simulink model "test_ps_helium_X"  (R2016a)
settings: Solver=VariableStepAuto  StartTime=0.0  StopTime=1000  RelTol=1e-3
libraries: simCryogenics_lib x18, nesl_utility x11
settings Model: Creator=FB229602  LastModifiedBy=FB229602
settings GRTTargetCC: GeneratePreprocessorConditionals=Use local settings
settings SimscapeCC: SimscapeLogType=all  SimscapeLogOpenViewer=on  SimscapeLogLimitData=off

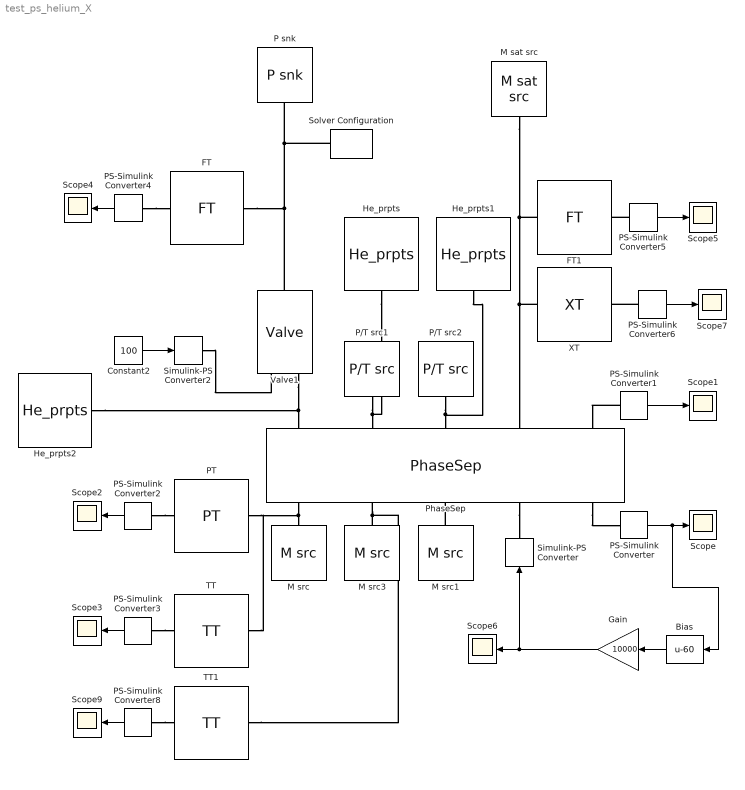
== system test_ps_helium_X ==
  Bias : Bias  Bias=-60
  Constant2 : Constant  Value=100
  FT : simCryogenics_lib/Sensors/FT
  FT1 : simCryogenics_lib/Sensors/FT
  Gain : Gain  Gain=10000
  He_prpts : simCryogenics_lib/Utilities/He_prpts  P_min=0.2 bar  T_min=1 K  T_max=100 K  P_max=50 bar  Mol=4.0026 * (10 ^ (- 3)) kg/mol
  He_prpts1 : simCryogenics_lib/Utilities/He_prpts  P_min=0.2 bar  T_min=1 K  T_max=100 K  P_max=50 bar  Mol=4.0026 * (10 ^ (- 3)) kg/mol
  He_prpts2 : simCryogenics_lib/Utilities/He_prpts  P_min=0.2 bar  T_min=1 K  T_max=100 K  P_max=50 bar  Mol=4.0026 * (10 ^ (- 3)) kg/mol
  M sat src : simCryogenics_lib/Sources_Sinks/M sat src  M=0.1 kg/s  Xmix=0.5
  M src : simCryogenics_lib/Sources_Sinks/M src  M=0 kg/s
  M src1 : simCryogenics_lib/Sources_Sinks/M src  M=0.05 kg/s
  M src3 : simCryogenics_lib/Sources_Sinks/M src  M=0.05 kg/s
  P snk : simCryogenics_lib/Sources_Sinks/P snk  P=1.05 bar
  P/T src1 : simCryogenics_lib/Sources_Sinks/P//T src  P=5 bar  T=5 K
  P/T src2 : simCryogenics_lib/Sources_Sinks/P//T src  P=5 bar  T=5 K
  PS-Simulink Converter{,1..6,8} (8 alike) : nesl_utility/PS-Simulink Converter  PhysicalDomain=network_engine_domain  SubClassName=ps_output  LeftPortType=input  RightPortType=output  PseudoPeriodic=off  Frequencies=[]  Unit=1  AffineConversion=off
  PT : simCryogenics_lib/Sensors/PT
  PhaseSep : simCryogenics_lib/Elements/PhaseSep  Ideal1=1  DeltaT1=0.05 K  N1=10  h1=400 W/K  Ideal2=1  DeltaT2=0.05 K  N2=10  h2=400 W/K  hmax=1.5 m  S=0.2 m^2  P0=1.2 bar  h0=62
  Scope{,1..7,9} (9 alike) : Scope
  Simulink-PS Converter : nesl_utility/Simulink-PS Converter  PhysicalDomain=network_engine_domain  SubClassName=ps_input  LeftPortType=input  RightPortType=output  PseudoPeriodic=off  Frequencies=[]  NoiseDistribution=none  NoiseParameters=[]  Unit=1  AffineConversion=off  InputFiltering=off  SimscapeFilterOrder=1  InputFilterTimeConstant=0.001  UdotUserProvided=1
  Simulink-PS Converter2 : nesl_utility/Simulink-PS Converter  PhysicalDomain=network_engine_domain  SubClassName=ps_input  LeftPortType=input  RightPortType=output  PseudoPeriodic=off  Frequencies=[]  NoiseDistribution=none  NoiseParameters=[]  Unit=1  AffineConversion=off  InputFiltering=off  SimscapeFilterOrder=1  InputFilterTimeConstant=0.001  UdotUserProvided=1
  Solver Configuration : nesl_utility/Solver Configuration  PhysicalDomain=network_engine_domain  SubClassName=solver  LeftPortType=input  RightPortType=generic  Accelerate=off  Tones=[]  Harmonics=[]  SimulateNoise=off  Profile=off  UseLocalSampling=off  EnableSwitchedLinearOptims=on  FrequencyDomain=off  UseCCode=off  RelTol=0.001  AbsTol=1e-06  MinStep=1e-09  ToWorkspace=off  RevertToSquareIcSolve=off  NumHomotopyIterations=100  PhasorMode=off  PhasorModeNumHarmonics=1  OverrideAbsTol=off  DoDC=off  ResidualTolerance=1e-09  UseLocalSolver=off  LocalSolverChoice=NE_BACKWARD_EULER_ADVANCER  LocalSolverSampleTime=0.001  DoFixedCost=off  MaxNonlinIter=3  MaxModeIter=2  LinearAlgebra=Sparse  DelaysMemoryBudget=1024  AutomaticFiltering=on  FilteringTimeConstant=0.001
  TT : simCryogenics_lib/Sensors/TT
  TT1 : simCryogenics_lib/Sensors/TT
  Valve1 : simCryogenics_lib/Elements/Valve  CVmax=100  ControlInputMin=0  ControlInputMax=100  Xt=0.86  Rv=10  lin_v=0  lim_v=0  K=2.4e-5 m^1.50000*kg^0.50000/s/bar^0.50000  Cmd_specify=off  Cmd_priority=None  Cmd=0  gamma_specify=off  gamma_priority=None  gamma=0  rho_specify=off  rho_priority=None  rho=0 kg/m^3  Xc_specify=off  Xc_priority=None  Xc=0  X_specify=off  X_priority=None  X=0  Y_specify=off  Y_priority=None  Y=0  CV_specify=off  CV_priority=None  CV=0
  XT : simCryogenics_lib/Sensors/XT
  wires:
  Gain/1 -> Simulink-PS Converter/1, Scope6/1
  PS-Simulink Converter/1 -> Bias/1, Scope/1
  PS-Simulink Converter1/1 -> Scope1/1
  Constant2/1 -> Simulink-PS Converter2/1
  PS-Simulink Converter2/1 -> Scope2/1
  PS-Simulink Converter3/1 -> Scope3/1
  PS-Simulink Converter4/1 -> Scope4/1
  PS-Simulink Converter5/1 -> Scope5/1
  Bias/1 -> Gain/1
  PS-Simulink Converter6/1 -> Scope7/1
  PS-Simulink Converter8/1 -> Scope9/1
  connections:
  PhaseSep/RConn1 -- TT/LConn1 -- PT/LConn1 -- M src/RConn1
  Valve1/RConn1 -- FT/LConn1 -- P snk/RConn1 -- Solver Configuration/RConn1
  FT1/LConn1 -- XT/LConn1 -- PhaseSep/LConn4 -- M sat src/RConn1
  M src3/RConn1 -- TT1/LConn1 -- PhaseSep/RConn2
  M src1/RConn1 -- PhaseSep/RConn3
  PhaseSep/RConn4 -- Simulink-PS Converter/RConn1
  PhaseSep/RConn5 -- PS-Simulink Converter/LConn1
  PS-Simulink Converter1/LConn1 -- PhaseSep/LConn5
  Valve1/LConn2 -- He_prpts2/RConn1 -- PhaseSep/LConn1
  Simulink-PS Converter2/RConn1 -- Valve1/LConn1
  PS-Simulink Converter2/LConn1 -- PT/RConn1
  P/T src1/RConn1 -- He_prpts/RConn1 -- PhaseSep/LConn2
  P/T src2/RConn1 -- He_prpts1/RConn1 -- PhaseSep/LConn3
  PS-Simulink Converter3/LConn1 -- TT/RConn1
  PS-Simulink Converter4/LConn1 -- FT/RConn1
  PS-Simulink Converter5/LConn1 -- FT1/RConn1
  PS-Simulink Converter6/LConn1 -- XT/RConn1
  PS-Simulink Converter8/LConn1 -- TT1/RConn1
